simulink model "transmission_estimation"  (R2016b)
settings: Solver=FixedStepDiscrete  StartTime=0.0  StopTime=inf  FixedStep=sampleTime  RelTol=1e-3
InitFcn:
  | model_affc_parameters;
StartFcn:
  | model_affc_parameters;
libraries: LibraryFM x4
settings Model: SimulationMode=external  Creator=niekbeckers  LastModifiedBy=Labuser
settings DataIOCC: LimitDataPoints=on  SaveFormat=Array
settings OptimizationCC: BlockReduction=off  BooleanDataType=off  LocalBlockOutputs=off  LifeSpan=inf
settings DebuggingCC: SaveWithParameterizedLinksMsg=none  UnderspecifiedInitializationDetection=Classic  MergeDetectMultiDrivingBlocksExec=none  SignalResolutionControl=TryResolveAllWithWarning  SFUnexpectedBacktrackingDiag=warning  SFNoUnconditionalDefaultTransitionDiag=warning  SFExecutionAtInitializationDiag=none
settings HardwareCC: ProdBitPerPointer=32  ProdBitPerSizeT=32  ProdBitPerPtrDiffT=32  ProdLargestAtomicFloat=None  ProdIntDivRoundTo=Undefined  ProdEndianess=Unspecified  ProdWordSize=32  ProdHWDeviceType=32-bit Generic  TargetBitPerPointer=64  TargetBitPerSizeT=64  TargetBitPerPtrDiffT=64  TargetLongLongMode=on  TargetIntDivRoundTo=Zero  TargetEndianess=LittleEndian  TargetWordSize=64  TargetHWDeviceType=MATLAB Host  ProdEqTarget=off
settings ModelReferenceCC: PropagateSignalLabelsOutOfModel=off
settings RTWCC: SystemTargetFile=TwinCAT.tlc  GenCodeOnly=on  MakeCommand=make_tct  TemplateMakefile=tct_msbuild.tmf  Description=TwinCAT Target  GenerateReport=on  TargetLang=C++
settings STFCustomTargetCC: CompOptLevelCompliant=on  GeneratePreprocessorConditionals=Disable all  MATLABClassNameForMDSCustomization=Simulink.SoftwareTarget.TargetSpecificTriggerConfigurationBase  SystemTargetFile=TwinCAT.tlc
settings ConfigComp: CovMetricSettings=dw  CovHtmlReporting=on  CovSaveCumulativeToWorkspaceVar=on  CovSaveSingleToWorkspaceVar=on  CovExternalEMLEnable=off  CovSFcnEnable=off

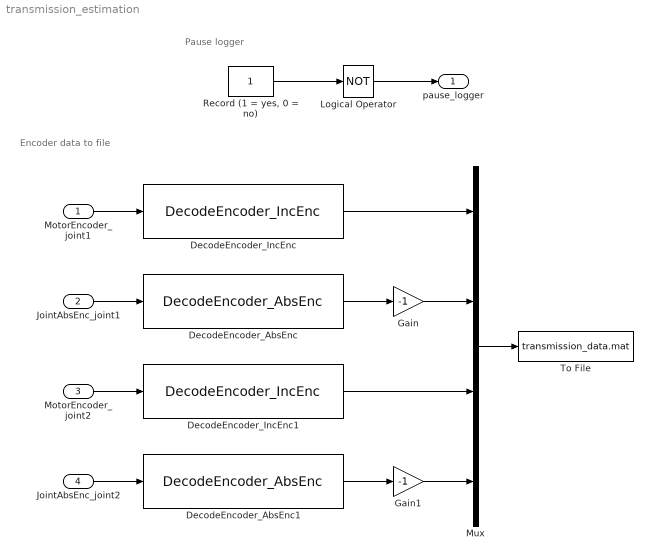
== system transmission_estimation ==
  note: Pause logger
  note: Encoder data to file
  MotorEncoder_joint1 : Inport  OutDataTypeStr=int32  PortDimensions=1
  JointAbsEnc_joint1 : Inport  Port=2  OutDataTypeStr=int32  PortDimensions=1
  MotorEncoder_joint2 : Inport  Port=3  OutDataTypeStr=int32  PortDimensions=1
  JointAbsEnc_joint2 : Inport  Port=4  OutDataTypeStr=int32  PortDimensions=1
  DecodeEncoder_AbsEnc : LibraryFM/FromActuator1/DecodeEncoder_AbsEnc  EncoderCounts_rev=FM1.Actuator1.JointAbsoluteEncoderCounts_rev
  DecodeEncoder_AbsEnc1 : LibraryFM/FromActuator1/DecodeEncoder_AbsEnc  EncoderCounts_rev=FM1.Actuator1.JointAbsoluteEncoderCounts_rev
  DecodeEncoder_IncEnc : LibraryFM/FromActuator1/DecodeEncoder_IncEnc  EncoderCounts_rev=FM1.Actuator1.MotorEncoderCounts_rev
  DecodeEncoder_IncEnc1 : LibraryFM/FromActuator1/DecodeEncoder_IncEnc  EncoderCounts_rev=FM1.Actuator2.MotorEncoderCounts_rev
  Gain : Gain  Gain=-1
  Gain1 : Gain  Gain=-1
  Logical Operator : Logic  Operator=NOT  Inputs=1  AllPortsSameDT=off  OutDataTypeStr=boolean
  Mux : Mux
  "Record (1 = yes, 0 = no)" : Constant  OutDataTypeStr=double
      settings: OpenFcn=|
      | b = get_param(gcb,'value');
      | if (strcmp(b,'1')),
      |   set_param (gcb,'value','0');
      | else
      |   set_param(gcb,'value','1');
      | end;
  To File : ToFile  Filename=transmission_data.mat  MatrixName=data
  pause_logger : Outport  OutDataTypeStr=boolean
  wires:
  Mux/1 -> To File/1
  MotorEncoder_joint1/1 -> DecodeEncoder_IncEnc/1
  JointAbsEnc_joint1/1 -> DecodeEncoder_AbsEnc/1
  MotorEncoder_joint2/1 -> DecodeEncoder_IncEnc1/1
  JointAbsEnc_joint2/1 -> DecodeEncoder_AbsEnc1/1
  "Record (1 = yes, 0 = no)"/1 -> Logical Operator/1
  Logical Operator/1 -> pause_logger/1
  DecodeEncoder_IncEnc/1 -> Mux/1
  DecodeEncoder_IncEnc1/1 -> Mux/3
  DecodeEncoder_AbsEnc/1 -> Gain/1
  DecodeEncoder_AbsEnc1/1 -> Gain1/1
  Gain/1 -> Mux/2
  Gain1/1 -> Mux/4
